simulink model "sampleModel1546"  (R2023a)
settings: Solver=VariableStepAuto  StartTime=0.0  StopTime=10.0  RelTol=1e-3
libraries: hdlsllib x2
settings Model: Creator=user1  LastModifiedBy=user1

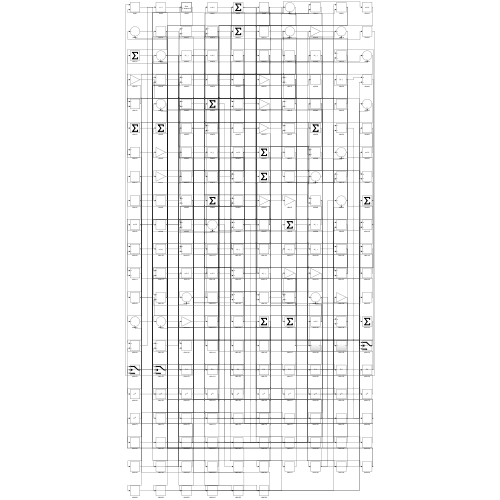
[thumbnail: Simulink's stored preview of the top-level diagram]
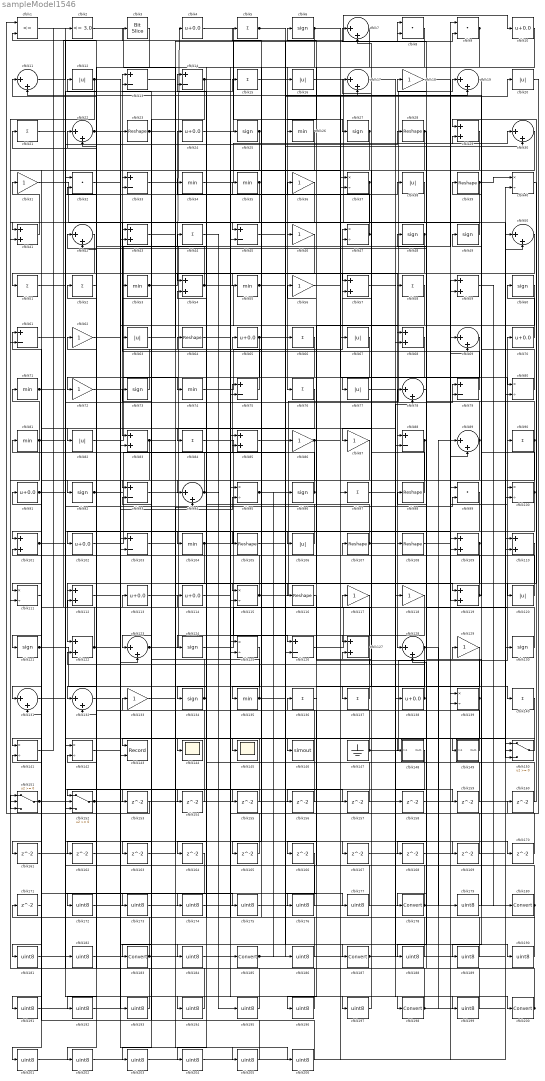
== system sampleModel1546 ==
  cfblk1 : RelationalOperator  Operator=<=  OutDataTypeStr=boolean  InputSameDT=off
  cfblk{4,10,24,65,70,91,102,113..114,138} (10 alike) : Bias  Bias=0.0  SaturateOnIntegerOverflow=off
  cfblk{37,40,47,80,95,100,111,115,125,139,141..142} (12 alike) : Product  Inputs=*/  RndMeth=Zero  SaturateOnIntegerOverflow=on
  cfblk{29,41,43,54,57,59,68,83,85,101,109..110,112,119,122,127} (16 alike) : Sum
  cfblk{13..14,33,45,61,75,79,88,93,103,126} (11 alike) : Sum  Inputs=+-
  cfblk{26,34..35,53,55,71,74,81,104,135} (10 alike) : MinMax
  cfblk{23,28,39,64,98,105,107..108,116} (9 alike) : Reshape
  cfblk{12,16,20,38,63,67,77,82,106,120} (10 alike) : Abs  SaturateOnIntegerOverflow=off
  cfblk{7,11,17,19,22,30,42,50,69,78,89,94,123,128,131..132} (16 alike) : Sum  Inputs=|++
  cfblk{18,31,36,46,56,62,72,86..87,117..118,129,133} (13 alike) : Gain
  cfblk{6,25,27,48..49,60,73,92,96,121,124,130,134} (13 alike) : Signum
  cfblk{5,15,21,44,51..52,58,66,76,84,90,97,136..137,140} (15 alike) : Sum  Inputs=+
  cfblk143 : Record  FileSettingsInternal="{\"entries\":[{\"content\":{\"excelSettings\":{\"content\":{},\"type\":\"Streamout.ExcelSettings\"}},\"type\":\"Streamout.FileSettingStorage\",\"uuid\":\"\"}],\"packageUris\":[\"http:\\/\\/schema.mathworks.com\\/mf0\\/streamout_blocks\\/R2020a\"],\"version\":\"1.0\"}"  Layout=[1 1]  SignalsInternal="{\"entries\":[{\"content\":{\"signals\":[{\"content\":{\"blockPath\":[],\"dimensions\":[1],\"domain\":\"\",\"lineColor\":\"#a2142f\",\"plots\":[1],\"port\":1,\"signalID\":1619,\"signalName\":\"XY Graph:1\"},\"type\":\"RecordBlkView.Signal\",\"uuid\":\"\"},{\"content\":{\"blockPath\":[],\"dimensions\":[1],\"domain\":\"\",\"lineColor\":\"#139fff\",\"plots\":[1],\"port\":2,\"signalID\":1622,\"signalName\":\"XY Graph:2\"},\"type\":\"RecordBlkView.Signal\",\"uuid\":\"\"}]},\"type\":\"RecordBlkView.InputSignals\",\"uuid\":\"\"}],\"packageUris\":[\"http:\\/\\/schema.mathworks.com\\/mf0\\/streamout_blocks\\/R2020a\"],\"version\":\"1.0\"}"  VisualizationBindings="{\"xyplotplugin\":{\"info\":[{\"series\":[{\"bindingParametersList\":[{\"parameter\":\"X-Axis\",\"signalID\":1619,\"signalName\":\"XY Graph:1\"},{\"parameter\":\"Y-Axis\",\"signalID\":1622,\"signalName\":\"XY Graph:2\"}],\"seriesID\":23041}],\"subplotID\":1}]}}"  CompatibilityTag=XY  st=-1
  cfblk144 : Scope
  cfblk145 : Scope
  cfblk146 : ToWorkspace  VariableName=simout  SaveFormat=Timeseries  SampleTime=-1
  cfblk147 : Ground
  cfblk148 : Subsystem
      settings: LibrarySourceBlock=|
      | hdlsllib/Ports &
      | Subsystems/Subsystem
  cfblk149 : Subsystem
      settings: LibrarySourceBlock=|
      | hdlsllib/Ports &
      | Subsystems/Subsystem
  cfblk150 : Switch  SaturateOnIntegerOverflow=off  InputSameDT=off
  cfblk151 : Switch  SaturateOnIntegerOverflow=off  InputSameDT=off
  cfblk152 : Switch  SaturateOnIntegerOverflow=off  InputSameDT=off
  cfblk{153..171} (19 alike) : Delay  SampleTime=1
  cfblk{172..177,179,181..182,184,186,188..197,199,201..206} (28 alike) : DataTypeConversion  OutDataTypeStr=uint8  SaturateOnIntegerOverflow=off  RndMeth=Floor
  cfblk{178,180,183,185,187,198,200} (7 alike) : DataTypeConversion  SaturateOnIntegerOverflow=off  RndMeth=Floor
  cfblk2 : hdlsllib/Logic and Bit Operations/Compare To Constant  relop=<=  const=3.0  OutDataTypeStr=boolean
  cfblk3 : hdlsllib/Logic and Bit Operations/Bit Slice  lidx=7  ridx=0
  cfblk{8..9,32,99} (4 alike) : DotProduct  OutDataTypeStr=Inherit: Inherit via internal rule
  wires:
  cfblk9/1 -> cfblk76/1, cfblk162/1
  cfblk34/1 -> cfblk30/1
  cfblk39/1 -> cfblk40/1, cfblk105/1
  cfblk135/1 -> cfblk113/1, cfblk169/1
  cfblk48/1 -> cfblk128/1, cfblk112/1
  cfblk12/1 -> cfblk151/3, cfblk184/1
  cfblk69/1 -> cfblk77/1
  cfblk107/1 -> cfblk5/1, cfblk199/1
  cfblk89/1 -> cfblk42/1, cfblk152/3
  cfblk141/1 -> cfblk2/1
  cfblk122/1 -> cfblk10/1, cfblk95/2
  cfblk147/1 -> cfblk70/1, cfblk42/2
  cfblk14/1 -> cfblk37/2, cfblk153/1
  cfblk53/1 -> cfblk4/1, cfblk68/2
  cfblk125/1 -> cfblk135/1
  cfblk115/1 -> cfblk19/1, cfblk8/2, cfblk101/2
  cfblk60/1 -> cfblk87/1
  cfblk47/1 -> cfblk24/1, cfblk137/1
  cfblk104/1 -> cfblk108/1, cfblk122/1
  cfblk138/1 -> cfblk6/1, cfblk35/1
  cfblk74/1 -> cfblk47/1
  cfblk139/1 -> cfblk7/1, cfblk155/1
  cfblk73/1 -> cfblk13/1
  cfblk152/1 -> cfblk29/1, cfblk139/2
  cfblk97/1 -> cfblk200/1
  cfblk95/1 -> cfblk38/1, cfblk186/1
  cfblk151/1 -> cfblk28/1, cfblk79/2
  cfblk99/1 -> cfblk102/1
  cfblk82/1 -> cfblk47/2
  cfblk35/1 -> cfblk45/1, cfblk93/1, cfblk51/1
  cfblk18/1 -> cfblk109/1
  cfblk23/1 -> cfblk145/1, cfblk115/2
  cfblk41/1 -> cfblk31/1
  cfblk16/1 -> cfblk150/1
  cfblk123/1 -> cfblk9/1, cfblk163/1
  cfblk68/1 -> cfblk106/1
  cfblk84/1 -> cfblk126/1
  cfblk25/1 -> cfblk54/1, cfblk75/2
  cfblk28/1 -> cfblk125/2, cfblk168/1
  cfblk126/1 -> cfblk90/1
  cfblk70/1 -> cfblk60/1
  cfblk54/1 -> cfblk88/1, cfblk21/1
  cfblk142/1 -> cfblk23/1
  cfblk80/1 -> cfblk11/2
  cfblk79/1 -> cfblk33/1
  cfblk72/1 -> cfblk74/1
  cfblk37/1 -> cfblk83/1, cfblk82/1, cfblk72/1
  cfblk27/1 -> cfblk84/1, cfblk61/2, cfblk173/1
  cfblk58/1 -> cfblk116/1
  cfblk102/1 -> cfblk16/1
  cfblk105/1 -> cfblk19/2
  cfblk101/1 -> cfblk36/1, cfblk161/1
  cfblk6/1 -> cfblk45/2, cfblk94/1, cfblk80/2, cfblk204/1
  cfblk26/1 -> cfblk55/1, cfblk43/2, cfblk141/1
  cfblk86/1 -> cfblk121/1, cfblk78/1
  cfblk22/1 -> cfblk68/1, cfblk123/2
  cfblk65/1 -> cfblk20/1, cfblk123/1, cfblk164/1
  cfblk134/1 -> cfblk63/1, cfblk114/1
  cfblk119/1 -> cfblk73/1, cfblk49/1
  cfblk38/1 -> cfblk41/1
  cfblk93/1 -> cfblk75/1
  cfblk31/1 -> cfblk69/1
  cfblk2/1 -> cfblk34/1
  cfblk150/1 -> cfblk143/1
  cfblk43/1 -> cfblk88/2
  cfblk128/1 -> cfblk146/1, cfblk179/1
  cfblk24/1 -> cfblk9/2
  cfblk149/1(Out1) -> cfblk54/2
  cfblk66/1 -> cfblk183/1
  cfblk59/1 -> cfblk180/1
  cfblk96/1 -> cfblk64/1, cfblk53/1
  cfblk88/1 -> cfblk143/2, cfblk148/1(In1)
  cfblk49/1 -> cfblk46/1
  cfblk98/1 -> cfblk17/1
  cfblk92/1 -> cfblk25/1, cfblk79/1
  cfblk44/1 -> cfblk185/1
  cfblk46/1 -> cfblk111/1
  cfblk55/1 -> cfblk86/1, cfblk170/1
  cfblk106/1 -> cfblk14/1
  cfblk10/1 -> cfblk124/1
  cfblk15/1 -> cfblk30/2
  cfblk11/1 -> cfblk3/1
  cfblk42/1 -> cfblk131/1
  cfblk137/1 -> cfblk56/1
  cfblk4/1 -> cfblk27/1
  cfblk130/1 -> cfblk98/1
  cfblk90/1 -> cfblk18/1, cfblk144/1
  cfblk113/1 -> cfblk115/1
  cfblk76/1 -> cfblk101/1
  cfblk129/1 -> cfblk178/1
  cfblk3/1 -> cfblk92/1
  cfblk132/1 -> cfblk150/2
  cfblk83/1 -> cfblk152/2, cfblk119/1
  cfblk124/1 -> cfblk69/2
  cfblk33/1 -> cfblk109/2
  cfblk120/1 -> cfblk107/1
  cfblk91/1 -> cfblk99/2, cfblk167/1
  cfblk64/1 -> cfblk126/2
  cfblk45/1 -> cfblk29/2
  cfblk13/1 -> cfblk58/1
  cfblk78/1 -> cfblk48/1
  cfblk62/1 -> cfblk198/1
  cfblk87/1 -> cfblk134/1
  cfblk61/1 -> cfblk15/1
  cfblk56/1 -> cfblk17/2
  cfblk71/1 -> cfblk194/1, cfblk201/1
  cfblk7/1 -> cfblk26/1
  cfblk127/1 -> cfblk61/1, cfblk122/2
  cfblk17/1 -> cfblk150/3
  cfblk1/1 -> cfblk104/1
  cfblk81/1 -> cfblk111/2, cfblk71/1, cfblk33/2
  cfblk57/1 -> cfblk80/1
  cfblk36/1 -> cfblk41/2
  cfblk52/1 -> cfblk132/1
  cfblk100/1 -> cfblk39/1, cfblk119/2
  cfblk30/1 -> cfblk57/1
  cfblk5/1 -> cfblk96/1, cfblk177/1
  cfblk110/1 -> cfblk127/1
  cfblk108/1 -> cfblk100/1
  cfblk121/1 -> cfblk140/1, cfblk175/1
  cfblk63/1 -> cfblk8/1
  cfblk75/1 -> cfblk43/1
  cfblk85/1 -> cfblk187/1
  cfblk51/1 -> cfblk149/1(In1)
  cfblk94/1 -> cfblk81/1, cfblk195/1
  cfblk40/1 -> cfblk120/1
  cfblk109/1 -> cfblk132/2, cfblk203/1
  cfblk153/1 -> cfblk1/1
  cfblk29/1 -> cfblk154/1
  cfblk154/1 -> cfblk1/2
  cfblk155/1 -> cfblk152/1
  cfblk148/1(Out1) -> cfblk156/1
  cfblk156/1 -> cfblk11/1
  cfblk21/1 -> cfblk157/1
  cfblk157/1 -> cfblk14/2
  cfblk158/1 -> cfblk139/1
  cfblk77/1 -> cfblk159/1
  cfblk159/1 -> cfblk37/1
  cfblk20/1 -> cfblk160/1
  cfblk160/1 -> cfblk127/2
  cfblk161/1 -> cfblk83/2
  cfblk162/1 -> cfblk22/2
  cfblk163/1 -> cfblk94/2
  cfblk8/1 -> cfblk165/1
  cfblk165/1 -> cfblk95/1
  cfblk116/1 -> cfblk166/1
  cfblk167/1 -> cfblk89/2
  cfblk168/1 -> cfblk40/2
  cfblk169/1 -> cfblk125/1
  cfblk170/1 -> cfblk7/2
  cfblk171/1 -> cfblk131/2
  cfblk67/1 -> cfblk172/1
  cfblk172/1 -> cfblk110/2
  cfblk173/1 -> cfblk67/1
  cfblk118/1 -> cfblk174/1
  cfblk174/1 -> cfblk110/1
  cfblk175/1 -> cfblk118/1
  cfblk136/1 -> cfblk176/1
  cfblk176/1 -> cfblk142/2
  cfblk177/1 -> cfblk136/1
  cfblk178/1 -> cfblk13/2, cfblk142/1
  cfblk179/1 -> cfblk129/1
  cfblk180/1 -> cfblk171/1, cfblk93/2, cfblk22/1
  cfblk166/1 -> cfblk181/1
  cfblk181/1 -> cfblk59/1
  cfblk131/1 -> cfblk182/1
  cfblk182/1 -> cfblk59/2
  cfblk183/1 -> cfblk141/2, cfblk100/2, cfblk52/1
  cfblk184/1 -> cfblk66/1
  cfblk185/1 -> cfblk78/2, cfblk138/1
  cfblk186/1 -> cfblk44/1
  cfblk187/1 -> cfblk158/1, cfblk57/2
  cfblk140/1 -> cfblk188/1
  cfblk188/1 -> cfblk85/1
  cfblk19/1 -> cfblk189/1
  cfblk189/1 -> cfblk85/2
  cfblk103/1 -> cfblk190/1
  cfblk190/1 -> cfblk65/1
  cfblk111/1 -> cfblk191/1
  cfblk191/1 -> cfblk103/1
  cfblk164/1 -> cfblk192/1
  cfblk192/1 -> cfblk103/2
  cfblk32/1 -> cfblk193/1
  cfblk193/1 -> cfblk151/1
  cfblk194/1 -> cfblk32/1
  cfblk195/1 -> cfblk32/2
  cfblk117/1 -> cfblk196/1
  cfblk196/1 -> cfblk12/1
  cfblk114/1 -> cfblk197/1
  cfblk197/1 -> cfblk117/1
  cfblk198/1 -> cfblk151/2, cfblk89/1, cfblk130/1
  cfblk199/1 -> cfblk62/1
  cfblk200/1 -> cfblk112/2, cfblk128/2
  cfblk201/1 -> cfblk97/1
  cfblk50/1 -> cfblk202/1
  cfblk202/1 -> cfblk99/1
  cfblk203/1 -> cfblk50/1
  cfblk204/1 -> cfblk50/2
  cfblk133/1 -> cfblk205/1
  cfblk205/1 -> cfblk91/1
  cfblk112/1 -> cfblk206/1
  cfblk206/1 -> cfblk133/1

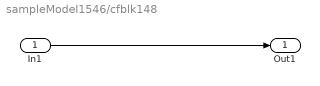
== system sampleModel1546/cfblk148 ==
  In1 : Inport
  Out1 : Outport
  wires:
  In1/1 -> Out1/1

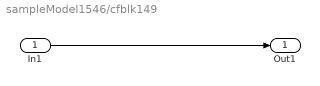
== system sampleModel1546/cfblk149 ==
  In1 : Inport
  Out1 : Outport
  wires:
  In1/1 -> Out1/1
